simulink model "MA4EE311Simu_5_2"  (R2019b)
settings: Solver=VariableStepAuto  StartTime=0.0  StopTime=10  RelTol=1e-3
libraries: dspsnks4 x1, dspsrcs4 x1, dspadpt3 x1
settings Model: Creator=hp  LastModifiedBy=hp

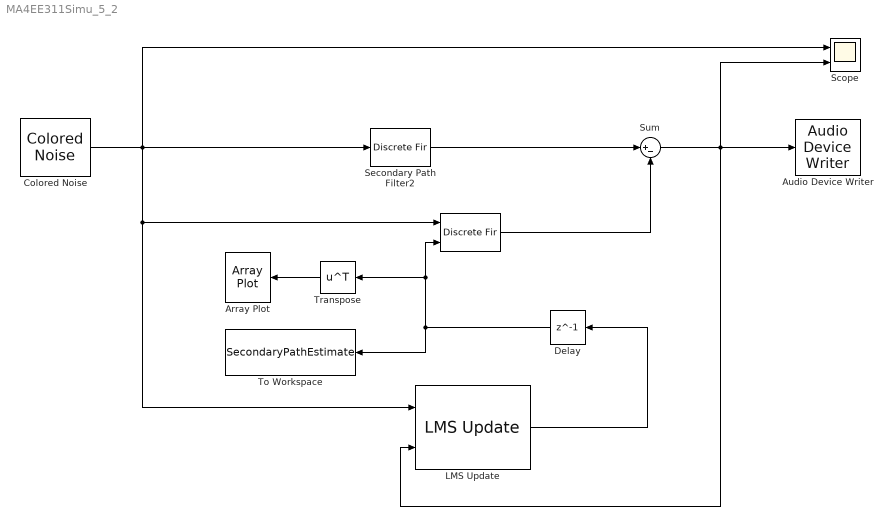
== system MA4EE311Simu_5_2 ==
  " " : DiscreteFir  CoefSource=Input port
      settings: InputPortMap=u0,u1
  Array Plot : ArrayPlot
  Audio Device Writer : dspsnks4/Audio Device Writer  Driver=DirectSound  Device=Default  InheritSampleRate=on  SampleRate=44100  BitDepth=16-bit integer  BufferSize=4096  NumBuffers=10  DefaultOutputChannelMapping=on  OutputChannelMapping=1:2  OutputNumUnderrunSamples=off  DriverIdx=1  DeviceWarnFlag=''
  Colored Noise : dspsrcs4/Colored Noise  Color=pink  InverseFrequencyPower=1  BoundedOutput=off  NumChannels=1  OutputDataType=double  SamplesPerFrame=1  SampleTime=1/4000  RandomStream=mt19937ar with seed  Seed=67  SimulateUsing=Interpreted execution
      settings: SourceProductName=DSP System Toolbox  SourceProductBaseCode=DS
  "Delay " : Delay  DelayLength=1  InitialCondition=0
  LMS Update : dspadpt3/LMS Update  Method=Normalized LMS  Length=32  StepSizeSource=Property  StepSize=0.01  LeakageFactor=1.0  InitialConditions=0  EnableAdaptInput=off  EnableResetInput=off  SimulateUsing=Code generation
      settings: SourceProductName=DSP System Toolbox  SourceProductBaseCode=DS
  Scope : Scope  NumInputPorts=2
  Secondary Path Filter2 : DiscreteFir  Coefficients=[ 0 0 -0.5 -0.5 -0.3 0.2 -0.1 0.5 -0.5 ]
  Sum : Sum  Inputs=|+-
  To Workspace : ToWorkspace  VariableName=SecondaryPathEstimate  SampleTime=1
      settings: Save2DSignal=2-D array (concatenate along first dimension)
  "Transpose " : Math  Operator=transpose  SignedPower=off  SaturateOnIntegerOverflow=on
  wires:
  "Delay "/1 -> To Workspace/1, "Transpose "/1, " "/2
  Secondary Path Filter2/1 -> Sum/1
  Sum/1 -> Scope/2, LMS Update/2, Audio Device Writer/1
  LMS Update/1 -> "Delay "/1
  " "/1 -> Sum/2
  Colored Noise/1 -> Scope/1, LMS Update/1, " "/1, Secondary Path Filter2/1
  "Transpose "/1 -> Array Plot/1
